simulink model "ol_rip_linandnonlin"  (R2019b)
settings: Solver=VariableStepAuto  StartTime=0.0  StopTime=10.0  RelTol=1e-3
values from neighbouring files (symbols this model uses):
  a = J+(m*r*r)    (= 0.028778125)    [ol_rip_linandnonlin_params.m]    (also in rotaryinvpend_params.m = 0.008078125)
  b = m*L*r    (= 0.0045015625)    [ol_rip_linandnonlin_params.m]    (also in rotaryinvpend_params.m)
  c = (4/3)*m*L*L    (= 0.00467604166667)    [ol_rip_linandnonlin_params.m]    (also in rotaryinvpend_params.m)
  d = m*g*L    (= 0.205396875)    [ol_rip_linandnonlin_params.m]    (also in rotaryinvpend_params.m)
  e = Beq+(nm*ng*kt*kg*kg*km)/rm    (= 0.0844985569231)    [ol_rip_linandnonlin_params.m]    (also in rotaryinvpend_params.m)
  f = (nm*ng*kt*kg)/rm    (= 0.151313076923)    [ol_rip_linandnonlin_params.m]    (also in rotaryinvpend_params.m)
  vm = 6    [ol_rip_linandnonlin_params.m]    (also in rotaryinvpend_params.m)
settings Model: Creator=SAI JOSHITHA  LastModifiedBy=SAI JOSHITHA

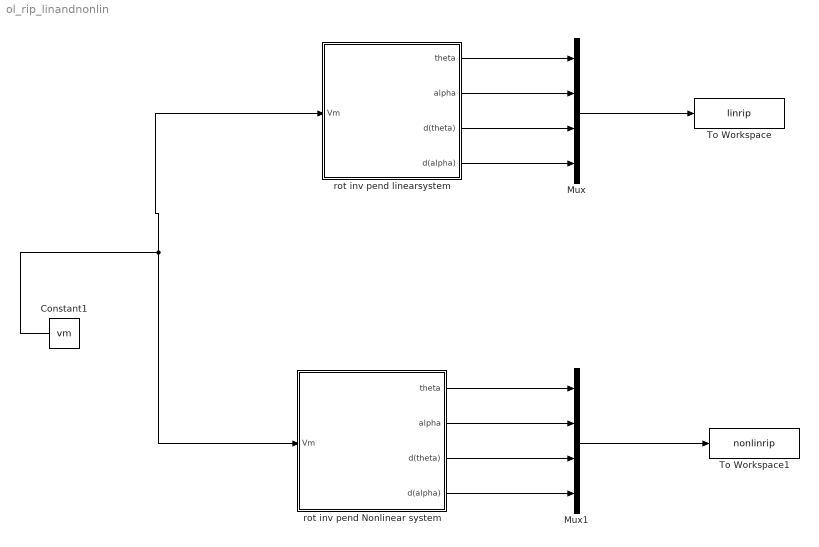
== system ol_rip_linandnonlin ==
  Constant1 : Constant  Value=vm
  Mux : Mux
  Mux1 : Mux
  To Workspace : ToWorkspace  VariableName=linrip  SaveFormat=Timeseries  SampleTime=-1
  To Workspace1 : ToWorkspace  VariableName=nonlinrip  SaveFormat=Timeseries  SampleTime=-1
  rot inv pend Nonlinear system : Subsystem
  rot inv pend linearsystem : Subsystem
  wires:
  rot inv pend linearsystem/1(theta) -> Mux/1
  Mux/1 -> To Workspace/1
  rot inv pend linearsystem/2(alpha) -> Mux/2
  rot inv pend linearsystem/4(d(alpha)) -> Mux/4
  Constant1/1 -> rot inv pend linearsystem/1(Vm), rot inv pend Nonlinear system/1(Vm)
  rot inv pend Nonlinear system/3(d(theta)) -> Mux1/3
  rot inv pend linearsystem/3(d(theta)) -> Mux/3
  Mux1/1 -> To Workspace1/1
  rot inv pend Nonlinear system/2(alpha) -> Mux1/2
  rot inv pend Nonlinear system/4(d(alpha)) -> Mux1/4
  rot inv pend Nonlinear system/1(theta) -> Mux1/1

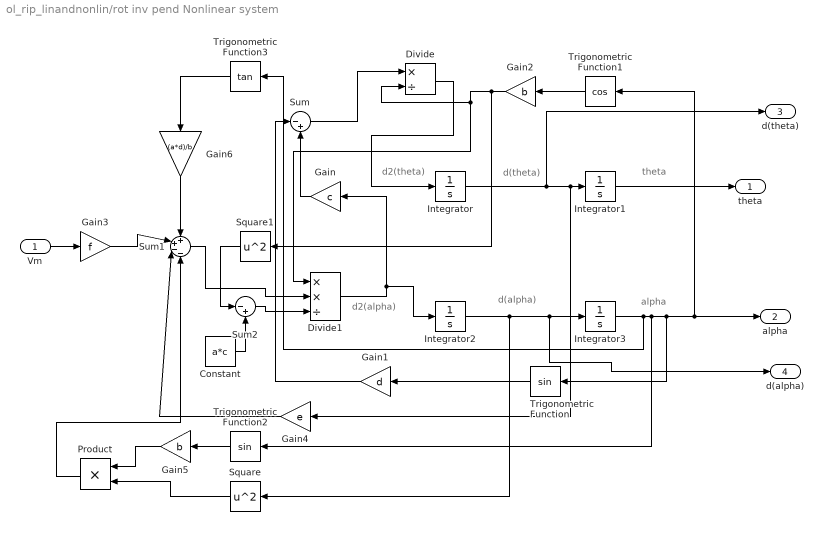
== system ol_rip_linandnonlin/rot inv pend Nonlinear system ==
  note: d2(alpha)
  note: d(alpha)
  note: alpha
  note: d2(theta)
  note: d(theta)
  note: theta
  Vm : Inport
  Constant : Constant  Value=a*c
  Divide : Product  Inputs=*/
  Divide1 : Product  Inputs=**/
  Gain : Gain  Gain=c
  Gain1 : Gain  Gain=d
  Gain2 : Gain  Gain=b
  Gain3 : Gain  Gain=f
  Gain4 : Gain  Gain=e
  Gain5 : Gain  Gain=b
  Gain6 : Gain  Gain=(a*d)/b
  Integrator{,1..3} (4 alike) : Integrator
  Product : Product
  Square : Math  Operator=square  SignedPower=off  SaturateOnIntegerOverflow=on
  Square1 : Math  Operator=square  SignedPower=off  SaturateOnIntegerOverflow=on
  Sum : Sum  Inputs=|-+
  Sum1 : Sum  Inputs=++--
  Sum2 : Sum  Inputs=|-+
  Trigonometric Function : Trigonometry
  Trigonometric Function1 : Trigonometry  Operator=cos
  Trigonometric Function2 : Trigonometry
  Trigonometric Function3 : Trigonometry  Operator=tan
  theta : Outport
  alpha : Outport  Port=2
  d(theta) : Outport  Port=3
  d(alpha) : Outport  Port=4
  wires:
  Vm/1 -> Gain3/1
  Integrator2/1 -> Square/1, Integrator3/1, d(alpha)/1
  Integrator/1 -> d(theta)/1, Gain4/1, Integrator1/1
  Integrator3/1 -> Trigonometric Function3/1, Trigonometric Function2/1, Trigonometric Function1/1, alpha/1, Trigonometric Function/1
  Integrator1/1 -> theta/1
  Gain/1 -> Sum/2
  Trigonometric Function/1 -> Gain1/1
  Gain1/1 -> Sum/1
  Trigonometric Function1/1 -> Gain2/1
  Sum/1 -> Divide/1
  Gain2/1 -> Square1/1, Divide1/1, Divide/2
  Divide/1 -> Integrator/1
  Gain3/1 -> Sum1/2
  Gain4/1 -> Sum1/3
  Trigonometric Function2/1 -> Gain5/1
  Gain5/1 -> Product/1
  Square/1 -> Product/2
  Product/1 -> Sum1/4
  Trigonometric Function3/1 -> Gain6/1
  Gain6/1 -> Sum1/1
  Divide1/1 -> Gain/1, Integrator2/1
  Square1/1 -> Sum2/1
  Sum1/1 -> Divide1/2
  Sum2/1 -> Divide1/3
  Constant/1 -> Sum2/2

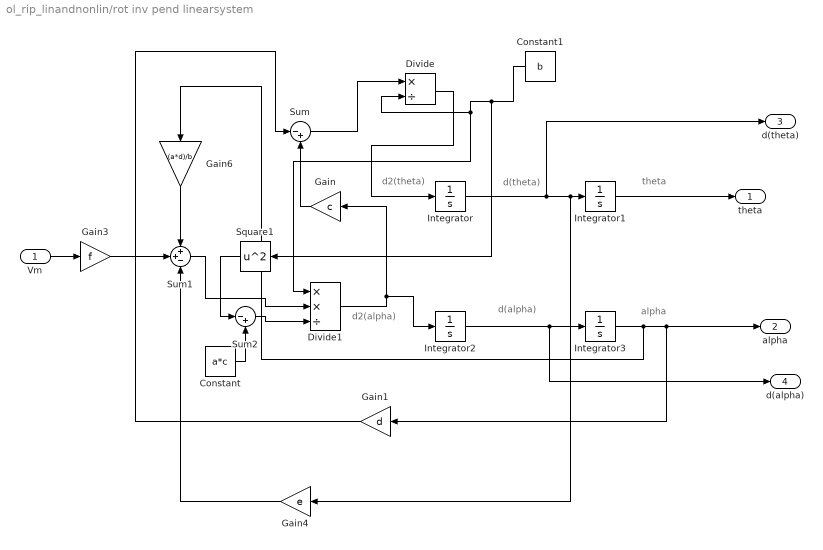
== system ol_rip_linandnonlin/rot inv pend linearsystem ==
  note: d2(theta)
  note: d(theta)
  note: alpha
  note: d2(alpha)
  note: d(alpha)
  note: theta
  Vm : Inport
  Constant : Constant  Value=a*c
  Constant1 : Constant  Value=b
  Divide : Product  Inputs=*/
  Divide1 : Product  Inputs=**/
  Gain : Gain  Gain=c
  Gain1 : Gain  Gain=d
  Gain3 : Gain  Gain=f
  Gain4 : Gain  Gain=e
  Gain6 : Gain  Gain=(a*d)/b
  Integrator{,1..3} (4 alike) : Integrator
  Square1 : Math  Operator=square  SignedPower=off  SaturateOnIntegerOverflow=on
  Sum : Sum  Inputs=|-+
  Sum1 : Sum  Inputs=++-
  Sum2 : Sum  Inputs=|-+
  theta : Outport
  alpha : Outport  Port=2
  d(theta) : Outport  Port=3
  d(alpha) : Outport  Port=4
  wires:
  Square1/1 -> Sum2/1
  Constant/1 -> Sum2/2
  Divide/1 -> Integrator/1
  Gain3/1 -> Sum1/2
  Sum2/1 -> Divide1/3
  Gain4/1 -> Sum1/3
  Constant1/1 -> Square1/1, Divide1/1, Divide/2
  Gain1/1 -> Sum/1
  Sum/1 -> Divide/1
  Divide1/1 -> Gain/1, Integrator2/1
  Sum1/1 -> Divide1/2
  Integrator1/1 -> theta/1
  Integrator2/1 -> Integrator3/1, d(alpha)/1
  Integrator/1 -> d(theta)/1, Gain4/1, Integrator1/1
  Vm/1 -> Gain3/1
  Integrator3/1 -> Gain6/1, Gain1/1, alpha/1
  Gain/1 -> Sum/2
  Gain6/1 -> Sum1/1
